simulink model "ACS"  (R2020a)
settings: Solver=VariableStepAuto  StartTime=0.0  StopTime=10.0  RelTol=1e-3
model workspace (MAT data in the model file):
  AccessStatus = Simulink.Bus
  AccessStatus.Alignment = -1
  AccessStatus.Elements_internal = Simulink.BusElement
  AccessStatus.Elements_internal.DimensionsMode = 'Fixed'
  AccessStatus.Elements_internal.SamplingMode = 'Sample based'
  AccessStatus.Elements_internal.SampleTime = -1
  AccessStatus.Elements_internal.Name = 'status'
  AccessStatus.Elements_internal.DataType_internal = 'boolean'
  AccessStatus.Elements_internal.Complexity = 'real'
  AccessStatus.Elements_internal.Dimensions = 1
  AccessStatus.DataScope = 'Auto'
settings Model: OrderedModelArguments=off  Creator=filaretovna  LastModifiedBy=filaretovna

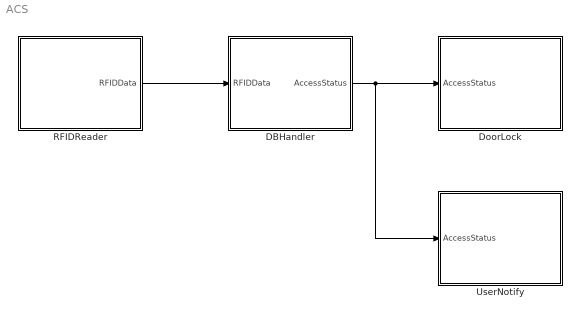
== system ACS ==
  DBHandler : Subsystem
      settings: PortSchema="{\"entries\":[{\"content\":{\"headerSize\":26,\"margin\":15,\"minimumSpacing\":25,\"sides\":[{\"content\":{\"connectorIds\":[\"In1\"]},\"type\":\"ConnectorPlacement.EquallySpacedRectSide\",\"uuid\":\"bf950cb8-06ec-48c8-8a21-df032232bae0\"},{\"content\":{\"connectorIds\":[\"Out1\"],\"side\":\"RIGHT\"},\"type\":\"ConnectorPlacement.EquallySpacedRectSide\",\"uuid\":\"3dfcef5c-fde3-4b2e-a4e8-bd284fef3a25\"},{\"content\":{\"connectorIds\":[],\"side\":\"TOP\"},\"type\":\"ConnectorPlacement.EquallySpacedRectSide\",\"uuid\":\"6051eec4-3de0-4d2d-a6b3-6a30505375f7\"}]},\"type\":\"ConnectorPlacement.EquallySpacedConnector\",\"uuid\":\"c3013dc8-f34f-4d7a-afd9-b37a00cfd673\"}],\"packageUris\":[\"http://schema.mathworks.com/mf0/Connector/19700101\"],\"version\":\"1.0\"}"
  DoorLock : Subsystem
      settings: PortSchema="{\"entries\":[{\"content\":{\"headerSize\":26,\"margin\":15,\"minimumSpacing\":25,\"sides\":[{\"content\":{\"connectorIds\":[\"In1\"]},\"type\":\"ConnectorPlacement.EquallySpacedRectSide\",\"uuid\":\"bf950cb8-06ec-48c8-8a21-df032232bae0\"},{\"content\":{\"connectorIds\":[],\"side\":\"RIGHT\"},\"type\":\"ConnectorPlacement.EquallySpacedRectSide\",\"uuid\":\"3dfcef5c-fde3-4b2e-a4e8-bd284fef3a25\"},{\"content\":{\"connectorIds\":[],\"side\":\"TOP\"},\"type\":\"ConnectorPlacement.EquallySpacedRectSide\",\"uuid\":\"6051eec4-3de0-4d2d-a6b3-6a30505375f7\"}]},\"type\":\"ConnectorPlacement.EquallySpacedConnector\",\"uuid\":\"c3013dc8-f34f-4d7a-afd9-b37a00cfd673\"}],\"packageUris\":[\"http://schema.mathworks.com/mf0/Connector/19700101\"],\"version\":\"1.0\"}"
  RFIDReader : Subsystem
      settings: PortSchema="{\"entries\":[{\"content\":{\"headerSize\":26,\"margin\":15,\"minimumSpacing\":25,\"sides\":[{\"content\":{\"connectorIds\":[]},\"type\":\"ConnectorPlacement.EquallySpacedRectSide\",\"uuid\":\"bf950cb8-06ec-48c8-8a21-df032232bae0\"},{\"content\":{\"connectorIds\":[\"Out1\"],\"side\":\"RIGHT\"},\"type\":\"ConnectorPlacement.EquallySpacedRectSide\",\"uuid\":\"3dfcef5c-fde3-4b2e-a4e8-bd284fef3a25\"},{\"content\":{\"connectorIds\":[],\"side\":\"TOP\"},\"type\":\"ConnectorPlacement.EquallySpacedRectSide\",\"uuid\":\"6051eec4-3de0-4d2d-a6b3-6a30505375f7\"}]},\"type\":\"ConnectorPlacement.EquallySpacedConnector\",\"uuid\":\"c3013dc8-f34f-4d7a-afd9-b37a00cfd673\"}],\"packageUris\":[\"http://schema.mathworks.com/mf0/Connector/19700101\"],\"version\":\"1.0\"}"
  UserNotify : Subsystem
      settings: PortSchema="{\"entries\":[{\"content\":{\"headerSize\":26,\"margin\":15,\"minimumSpacing\":25,\"sides\":[{\"content\":{\"connectorIds\":[\"In1\"]},\"type\":\"ConnectorPlacement.EquallySpacedRectSide\",\"uuid\":\"bf950cb8-06ec-48c8-8a21-df032232bae0\"},{\"content\":{\"connectorIds\":[],\"side\":\"RIGHT\"},\"type\":\"ConnectorPlacement.EquallySpacedRectSide\",\"uuid\":\"3dfcef5c-fde3-4b2e-a4e8-bd284fef3a25\"},{\"content\":{\"connectorIds\":[],\"side\":\"TOP\"},\"type\":\"ConnectorPlacement.EquallySpacedRectSide\",\"uuid\":\"6051eec4-3de0-4d2d-a6b3-6a30505375f7\"}]},\"type\":\"ConnectorPlacement.EquallySpacedConnector\",\"uuid\":\"c3013dc8-f34f-4d7a-afd9-b37a00cfd673\"}],\"packageUris\":[\"http://schema.mathworks.com/mf0/Connector/19700101\"],\"version\":\"1.0\"}"
  wires:
  RFIDReader/1(RFIDData) -> DBHandler/1(RFIDData)
  DBHandler/1(AccessStatus) -> UserNotify/1(AccessStatus), DoorLock/1(AccessStatus)

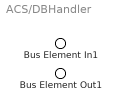
== system ACS/DBHandler ==
  Bus Element In1 : Inport  PortName=RFIDData
  Bus Element Out1 : Outport  PortName=AccessStatus

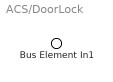
== system ACS/DoorLock ==
  Bus Element In1 : Inport  PortName=AccessStatus

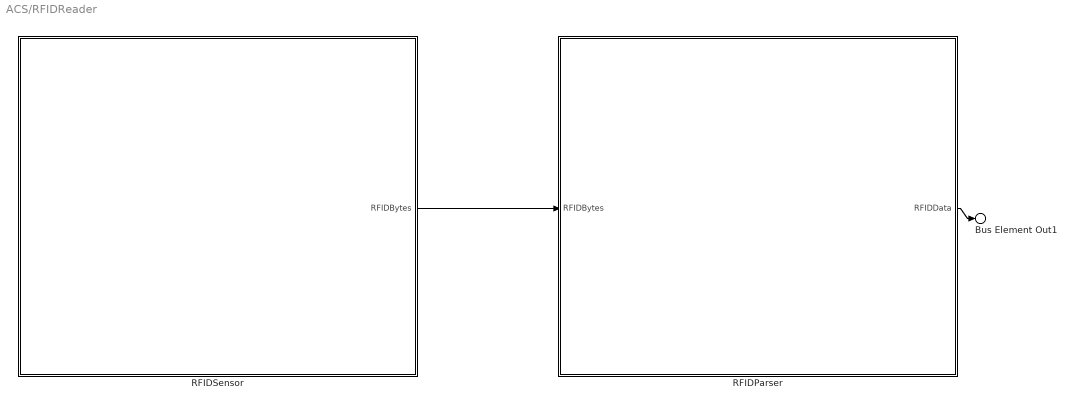
== system ACS/RFIDReader ==
  RFIDParser : Subsystem
      settings: PortSchema="{\"entries\":[{\"content\":{\"headerSize\":26,\"margin\":15,\"minimumSpacing\":25,\"sides\":[{\"content\":{\"connectorIds\":[\"In1\"]},\"type\":\"ConnectorPlacement.EquallySpacedRectSide\",\"uuid\":\"bf950cb8-06ec-48c8-8a21-df032232bae0\"},{\"content\":{\"connectorIds\":[\"Out1\"],\"side\":\"RIGHT\"},\"type\":\"ConnectorPlacement.EquallySpacedRectSide\",\"uuid\":\"3dfcef5c-fde3-4b2e-a4e8-bd284fef3a25\"},{\"content\":{\"connectorIds\":[],\"side\":\"TOP\"},\"type\":\"ConnectorPlacement.EquallySpacedRectSide\",\"uuid\":\"6051eec4-3de0-4d2d-a6b3-6a30505375f7\"}]},\"type\":\"ConnectorPlacement.EquallySpacedConnector\",\"uuid\":\"c3013dc8-f34f-4d7a-afd9-b37a00cfd673\"}],\"packageUris\":[\"http://schema.mathworks.com/mf0/Connector/19700101\"],\"version\":\"1.0\"}"
  RFIDSensor : Subsystem
      settings: PortSchema="{\"entries\":[{\"content\":{\"headerSize\":26,\"margin\":15,\"minimumSpacing\":25,\"sides\":[{\"content\":{\"connectorIds\":[]},\"type\":\"ConnectorPlacement.EquallySpacedRectSide\",\"uuid\":\"bf950cb8-06ec-48c8-8a21-df032232bae0\"},{\"content\":{\"connectorIds\":[\"Out1\"],\"side\":\"RIGHT\"},\"type\":\"ConnectorPlacement.EquallySpacedRectSide\",\"uuid\":\"3dfcef5c-fde3-4b2e-a4e8-bd284fef3a25\"},{\"content\":{\"connectorIds\":[],\"side\":\"TOP\"},\"type\":\"ConnectorPlacement.EquallySpacedRectSide\",\"uuid\":\"6051eec4-3de0-4d2d-a6b3-6a30505375f7\"}]},\"type\":\"ConnectorPlacement.EquallySpacedConnector\",\"uuid\":\"c3013dc8-f34f-4d7a-afd9-b37a00cfd673\"}],\"packageUris\":[\"http://schema.mathworks.com/mf0/Connector/19700101\"],\"version\":\"1.0\"}"
  Bus Element Out1 : Outport  PortName=RFIDData
  wires:
  RFIDSensor/1(RFIDBytes) -> RFIDParser/1(RFIDBytes)
  RFIDParser/1(RFIDData) -> Bus Element Out1/1

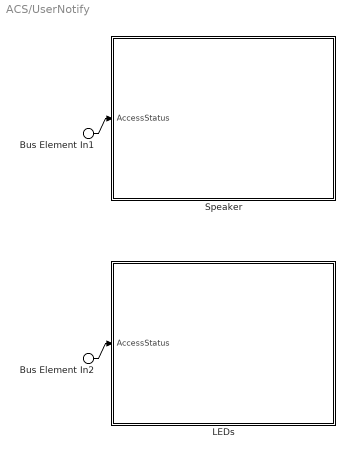
== system ACS/UserNotify ==
  Bus Element In1 : Inport  PortName=AccessStatus
  Bus Element In2 : Inport  PortName=AccessStatus
  LEDs : Subsystem
      settings: PortSchema="{\"entries\":[{\"content\":{\"headerSize\":26,\"margin\":15,\"minimumSpacing\":25,\"sides\":[{\"content\":{\"connectorIds\":[\"In1\"]},\"type\":\"ConnectorPlacement.EquallySpacedRectSide\",\"uuid\":\"bf950cb8-06ec-48c8-8a21-df032232bae0\"},{\"content\":{\"connectorIds\":[],\"side\":\"RIGHT\"},\"type\":\"ConnectorPlacement.EquallySpacedRectSide\",\"uuid\":\"3dfcef5c-fde3-4b2e-a4e8-bd284fef3a25\"},{\"content\":{\"connectorIds\":[],\"side\":\"TOP\"},\"type\":\"ConnectorPlacement.EquallySpacedRectSide\",\"uuid\":\"6051eec4-3de0-4d2d-a6b3-6a30505375f7\"}]},\"type\":\"ConnectorPlacement.EquallySpacedConnector\",\"uuid\":\"c3013dc8-f34f-4d7a-afd9-b37a00cfd673\"}],\"packageUris\":[\"http://schema.mathworks.com/mf0/Connector/19700101\"],\"version\":\"1.0\"}"
  Speaker : Subsystem
      settings: PortSchema="{\"entries\":[{\"content\":{\"headerSize\":26,\"margin\":15,\"minimumSpacing\":25,\"sides\":[{\"content\":{\"connectorIds\":[\"In1\"]},\"type\":\"ConnectorPlacement.EquallySpacedRectSide\",\"uuid\":\"bf950cb8-06ec-48c8-8a21-df032232bae0\"},{\"content\":{\"connectorIds\":[],\"side\":\"RIGHT\"},\"type\":\"ConnectorPlacement.EquallySpacedRectSide\",\"uuid\":\"3dfcef5c-fde3-4b2e-a4e8-bd284fef3a25\"},{\"content\":{\"connectorIds\":[],\"side\":\"TOP\"},\"type\":\"ConnectorPlacement.EquallySpacedRectSide\",\"uuid\":\"6051eec4-3de0-4d2d-a6b3-6a30505375f7\"}]},\"type\":\"ConnectorPlacement.EquallySpacedConnector\",\"uuid\":\"c3013dc8-f34f-4d7a-afd9-b37a00cfd673\"}],\"packageUris\":[\"http://schema.mathworks.com/mf0/Connector/19700101\"],\"version\":\"1.0\"}"
  wires:
  Bus Element In1/1 -> Speaker/1(AccessStatus)
  Bus Element In2/1 -> LEDs/1(AccessStatus)

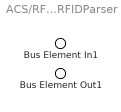
== system ACS/RFIDReader/RFIDParser ==
  Bus Element In1 : Inport  PortName=RFIDBytes
  Bus Element Out1 : Outport  PortName=RFIDData

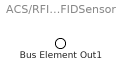
== system ACS/RFIDReader/RFIDSensor ==
  Bus Element Out1 : Outport  PortName=RFIDBytes

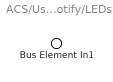
== system ACS/UserNotify/LEDs ==
  Bus Element In1 : Inport  PortName=AccessStatus

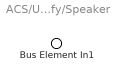
== system ACS/UserNotify/Speaker ==
  Bus Element In1 : Inport  PortName=AccessStatus
